simulink model "total_rocketmodel"  (R2023a)
settings: Solver=VariableStepAuto  StartTime=0.0  StopTime=10.0  RelTol=1e-3
values from neighbouring files (symbols this model uses):
  D = 0    [rocket_model.m]    (also in ss_model.mat; verif.m)
  g = 9.8    [main_rocketmodel.m]    (also in main_sim_rocket.m; rocket_model.m; sim_lin.m; test_bangbang.m)
  J_T = 40267    [main_rocketmodel.m]    (also in main_sim_rocket.m; rocket_model.m = 10)
  K_z = tf(lqg_ss)    [rocket_controllerdesign_z.m]
  m = 549054    [main_rocketmodel.m]    (also in main_sim_rocket.m; rocket_model.m = 25.4; sim_lin.m; test_bangbang.m)
  opt_controller = K_controller{k_min}    [main_yp_fminunc.m]    (also in reinforce_optim.m = s0_r0)
  sys = ss(A,B,C,D)    [controller_design.m]    (also in main_yp_fminunc.m; rocket_controllerdesign.m; rocket_controllerdesign_z.m; rocket_model.m)
  t_on = 14.6    [main_rocketmodel.m]    (also in main_sim_rocket.m; test_bangbang.m)
  Ts = 0.001    [main_rocketmodel.m]    (also in main_sim_rocket.m; sim_lin.m; square_sig.m; sum_squares_sig.m)
  x_0 = 0    [main_rocketmodel.m]    (also in main_sim_rocket.m)
  z_0 = 4000    [main_rocketmodel.m]    (also in main_sim_rocket.m; sim_lin.m; test_bangbang.m)
libraries: simulink x3
settings Model: Creator=bia  LastModifiedBy=bia
settings SolverCC: AlgebraicLoopSolver=TrustRegion
settings DataIOCC: ExternalInput=[t, Fe]
settings DebuggingCC: UnconnectedInputMsg=warning  UnconnectedOutputMsg=warning  UnconnectedLineMsg=warning
settings ModelReferenceCC: EnableRefExpFcnMdlSchedulingChecks=on

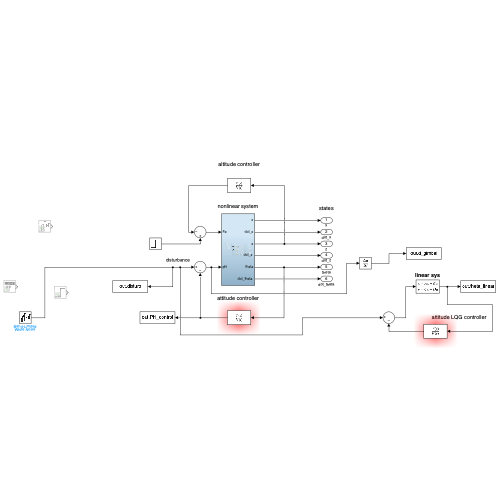
[thumbnail: Simulink's stored preview of the top-level diagram]
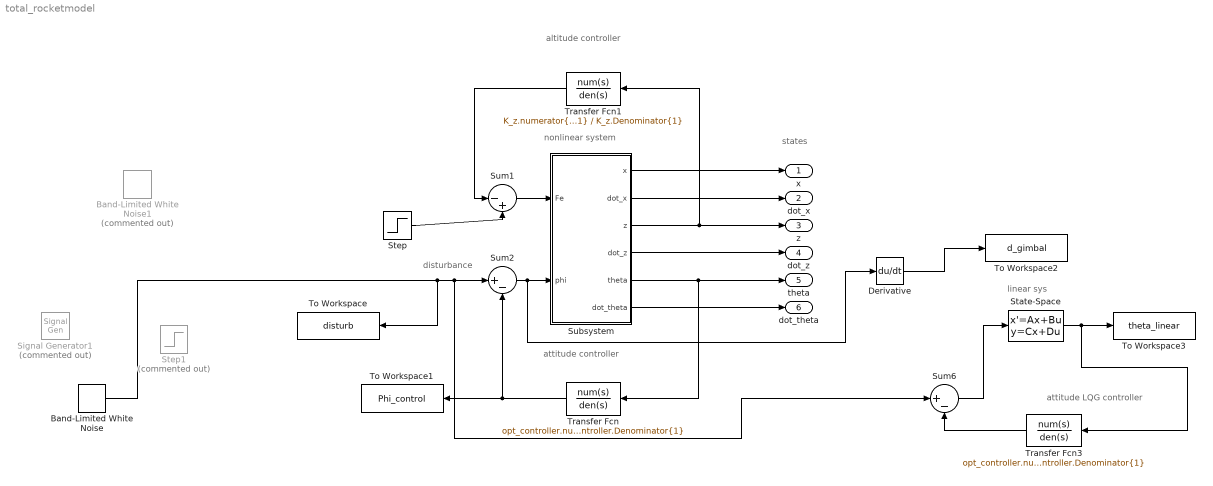
== system total_rocketmodel ==
  note: altitude controller
  note: attitude controller
  note: states
  note: disturbance
  note: nonlinear system
  note: attitude LQG controller
  note: linear sys
  Band-Limited White Noise : simulink/Sources/Band-Limited White Noise  Cov=1e-3  Ts=1  seed=[23341]
  Band-Limited White Noise1 : simulink/Sources/Band-Limited White Noise  Commented=on  Cov=1e-10  Ts=1  seed=[23341]
  Derivative : Derivative
  Signal Generator1 : SignalGenerator  Commented=on  WaveForm=square  Amplitude=1e-6  Units=rad/sec
  State-Space : StateSpace  A=sys.A  B=sys.B  C=sys.C  D=D  InitialCondition=0
  Step : Step  Time=t_on  Before=0.05*7e6  After=7e6  SampleTime=0
  Step1 : Step  Commented=on  Time=20  After=1e-4  SampleTime=Ts
  Subsystem : Subsystem
  Sum1 : Sum  Inputs=|-+
  Sum2 : Sum  Inputs=|+-
  Sum6 : Sum  Inputs=|+-
  To Workspace : ToWorkspace  VariableName=disturb  SampleTime=Ts
  To Workspace1 : ToWorkspace  VariableName=Phi_control  SampleTime=Ts
  To Workspace2 : ToWorkspace  VariableName=d_gimbal  SampleTime=Ts
  To Workspace3 : ToWorkspace  VariableName=theta_linear  SampleTime=Ts
  Transfer Fcn : TransferFcn  Numerator=opt_controller.numerator{1}  Denominator=opt_controller.Denominator{1}
  Transfer Fcn1 : TransferFcn  Numerator=K_z.numerator{1}  Denominator=K_z.Denominator{1}
  Transfer Fcn3 : TransferFcn  Numerator=opt_controller.numerator{1}  Denominator=opt_controller.Denominator{1}
  x : Outport
  "dot_x " : Outport  Port=2
  z : Outport  Port=3
  dot_z : Outport  Port=4
  theta : Outport  Port=5
  "dot_theta " : Outport  Port=6
  wires:
  Subsystem/1(x) -> x/1
  Subsystem/2(dot_x) -> "dot_x "/1
  Sum2/1 -> Derivative/1, Subsystem/2(phi)
  Subsystem/6("dot_theta ") -> "dot_theta "/1
  Subsystem/5(theta) -> Transfer Fcn/1, theta/1
  Subsystem/4("dot_z ") -> dot_z/1
  Subsystem/3(z) -> Transfer Fcn1/1, z/1
  Step/1 -> Sum1/2
  Transfer Fcn/1 -> Sum2/2, To Workspace1/1
  Sum1/1 -> Subsystem/1(Fe)
  Transfer Fcn1/1 -> Sum1/1
  Band-Limited White Noise/1 -> To Workspace/1, Sum6/1, Sum2/1
  State-Space/1 -> Transfer Fcn3/1, To Workspace3/1
  Transfer Fcn3/1 -> Sum6/2
  Sum6/1 -> State-Space/1
  Derivative/1 -> To Workspace2/1

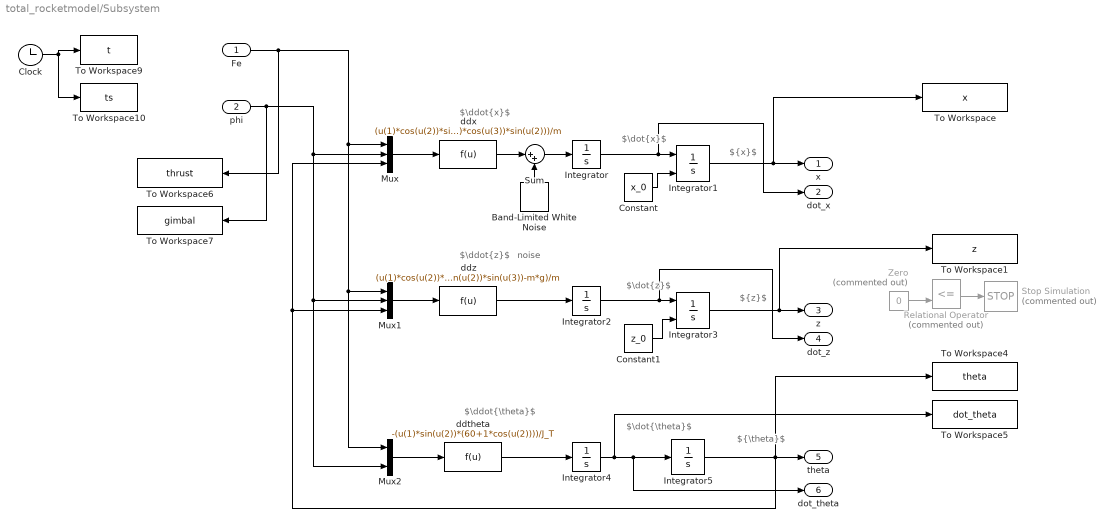
== system total_rocketmodel/Subsystem ==
  note: $\dot{z}$
  note: $\ddot{z}$
  note: ${z}$
  note: $\ddot{\theta}$
  note: $\ddot{x}$
  note: $\dot{x}$
  note: $\dot{\theta}$
  note: ${x}$
  note: ${\theta}$
  note: noise
  Fe : Inport
  phi : Inport  Port=2
  Band-Limited White Noise : simulink/Sources/Band-Limited White Noise  Cov=0  Ts=1  seed=[23341]
  Clock : Clock
  Constant : Constant  Value=x_0  SampleTime=Ts
  Constant1 : Constant  Value=z_0  SampleTime=Ts
  Integrator : Integrator  ContinuousStateAttributes='x_dot'
  Integrator1 : Integrator  InitialConditionSource=external  ContinuousStateAttributes='x'
  Integrator2 : Integrator  ContinuousStateAttributes='z_dot'
  Integrator3 : Integrator  InitialConditionSource=external  InitialCondition=50  LimitOutput=on  LowerSaturationLimit=0  ContinuousStateAttributes='z'
  Integrator4 : Integrator  ContinuousStateAttributes='theta_dot'
  Integrator5 : Integrator
  Mux : Mux  Inputs=3
  Mux1 : Mux  Inputs=3
  Mux2 : Mux  Inputs=2
  Relational Operator : RelationalOperator  Commented=on  Operator=<=  OutDataTypeStr=boolean  InputSameDT=off
  Stop Simulation : Stop  Commented=on
  Sum : Sum  Inputs=|++
  To Workspace : ToWorkspace  VariableName=x  SampleTime=Ts
  To Workspace1 : ToWorkspace  VariableName=z  SampleTime=Ts
  To Workspace10 : ToWorkspace  VariableName=ts  SampleTime=Ts
  To Workspace4 : ToWorkspace  VariableName=theta  SampleTime=Ts
  To Workspace5 : ToWorkspace  VariableName=dot_theta  SampleTime=Ts
  To Workspace6 : ToWorkspace  VariableName=thrust  SampleTime=Ts
  To Workspace7 : ToWorkspace  VariableName=gimbal  SampleTime=Ts
  To Workspace9 : ToWorkspace  VariableName=t  SampleTime=-1
  Zero : Constant  Commented=on  Value=0  OutDataTypeStr=Inherit: Inherit via back propagation
  ddtheta : Fcn  Expr=-(u(1)*sin(u(2))*(60+1*cos(u(2))))/J_T
  ddx : Fcn  Expr=(u(1)*cos(u(2))*sin(u(3))+u(1)*cos(u(3))*sin(u(2)))/m
  ddz : Fcn  Expr=(u(1)*cos(u(2))*cos(u(3))-u(1)*sin(u(2))*sin(u(3))-m*g)/m
  x : Outport
  dot_x : Outport  Port=2
  z : Outport  Port=3
  "dot_z " : Outport  Port=4
  theta : Outport  Port=5
  "dot_theta " : Outport  Port=6
  wires:
  ddtheta/1 -> Integrator4/1
  Mux/1 -> ddx/1
  Integrator2/1 -> "dot_z "/1, Integrator3/1
  Mux2/1 -> ddtheta/1
  Fe/1 -> To Workspace6/1, Mux2/1, Mux1/1, Mux/1
  Mux1/1 -> ddz/1
  Integrator/1 -> dot_x/1, Integrator1/1
  phi/1 -> To Workspace7/1, Mux2/2, Mux1/2, Mux/2
  Integrator3/1 -> z/1, To Workspace1/1
  Integrator5/1 -> To Workspace4/1, Mux1/3, Mux/3, theta/1
  Constant1/1 -> Integrator3/2
  Constant/1 -> Integrator1/2
  Integrator4/1 -> Integrator5/1, "dot_theta "/1, To Workspace5/1
  Integrator1/1 -> To Workspace/1, x/1
  Zero/1 -> Relational Operator/2
  Relational Operator/1 -> Stop Simulation/1
  Clock/1 -> To Workspace9/1, To Workspace10/1
  ddz/1 -> Integrator2/1
  Band-Limited White Noise/1 -> Sum/2
  ddx/1 -> Sum/1
  Sum/1 -> Integrator/1
